simulink model "SimulinkCircuitoRLC"  (R2023b)
settings: Solver=ode23s  StartTime=0.0  StopTime=0.0005  RelTol=1e-3
values from neighbouring files (symbols this model uses):
  C = 0.1e-6    (= 1e-07)    [CircuitoRLC.m]    (also in RLCparameters.mat)
  L = 4e-3    (= 0.004)    [CircuitoRLC.m]    (also in RLCparameters.mat)
  R = 120    [CircuitoRLC.m]    (also in RLCparameters.mat)

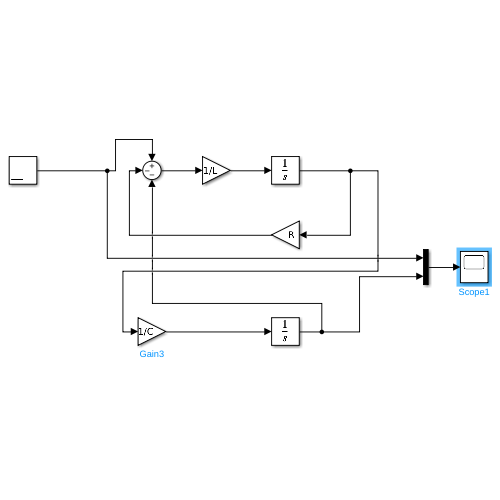
[thumbnail: Simulink's stored preview of the top-level diagram]
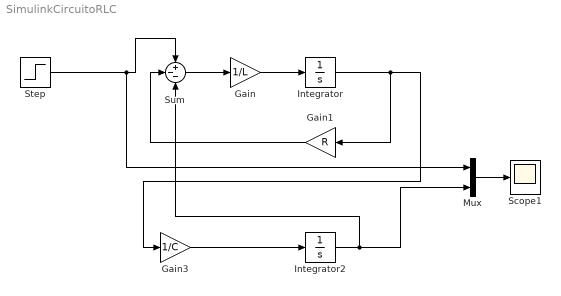
== system SimulinkCircuitoRLC ==
  Gain : Gain  Gain=1/L
  Gain1 : Gain  Gain=R
  Gain3 : Gain  Gain=1/C
  Integrator : Integrator
  Integrator2 : Integrator
  Mux : Mux  Inputs=2
  Scope1 : Scope
  Step : Step  Time=0  After=12  SampleTime=0
  Sum : Sum  Inputs=+--
  wires:
  Gain1/1 -> Sum/2
  Sum/1 -> Gain/1
  Gain/1 -> Integrator/1
  Step/1 -> Mux/1, Sum/1
  Gain3/1 -> Integrator2/1
  Mux/1 -> Scope1/1
  Integrator2/1 -> Mux/2, Sum/3
  Integrator/1 -> Gain3/1, Gain1/1
